simulink model "End_Angle_verification"  (R2019b)
settings: Solver=VariableStepAuto  StartTime=0.0  StopTime=10.0  RelTol=1e-3
values from neighbouring files (symbols this model uses):
  phi_d = zeros(N,1)    [parameters.m]
  phi_p = zeros(N,1)    [parameters.m]
settings Model: Creator=zceeash  LastModifiedBy=zceeash

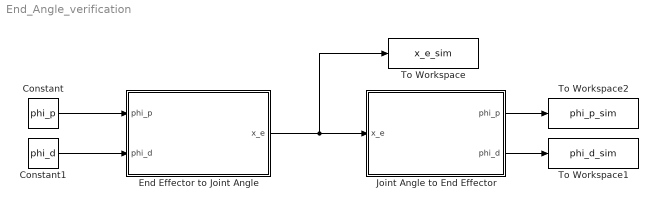
== system End_Angle_verification ==
  Constant : Constant  Value=phi_p
  Constant1 : Constant  Value=phi_d
  End Effector to Joint Angle : Subsystem
  Joint Angle to End Effector : Subsystem
  To Workspace : ToWorkspace  VariableName=x_e_sim  SaveFormat=Timeseries  SampleTime=-1
  To Workspace1 : ToWorkspace  VariableName=phi_d_sim  SaveFormat=Timeseries  SampleTime=-1
  To Workspace2 : ToWorkspace  VariableName=phi_p_sim  SaveFormat=Timeseries  SampleTime=-1
  wires:
  End Effector to Joint Angle/1(x_e) -> To Workspace/1, Joint Angle to End Effector/1(x_e)
  Joint Angle to End Effector/1(phi_p) -> To Workspace2/1
  Joint Angle to End Effector/2(phi_d) -> To Workspace1/1
  Constant/1 -> End Effector to Joint Angle/1(phi_p)
  Constant1/1 -> End Effector to Joint Angle/2(phi_d)

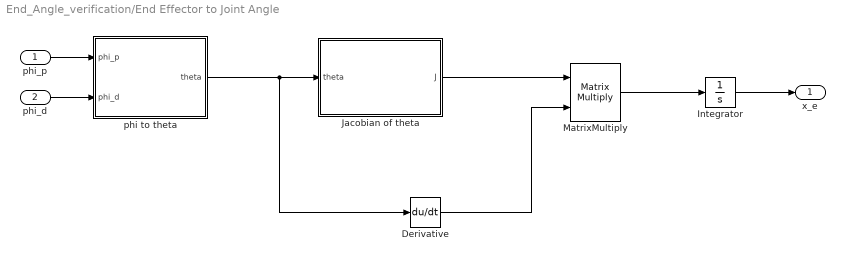
== system End_Angle_verification/End Effector to Joint Angle ==
  phi_p : Inport
  phi_d : Inport  Port=2
  Derivative : Derivative  CoefficientInTFapproximation=0
  Integrator : Integrator
  "Jacobian of theta " : MATLAB Function  TreatAsAtomicUnit=on
  MatrixMultiply : Product  Multiplication=Matrix(*)
  phi to theta : MATLAB Function  TreatAsAtomicUnit=on
  x_e : Outport
  wires:
  phi_p/1 -> phi to theta/1(phi_p)
  phi_d/1 -> phi to theta/2(phi_d)
  phi to theta/1(theta) -> Derivative/1, "Jacobian of theta "/1(theta)
  "Jacobian of theta "/1(J) -> MatrixMultiply/1
  Derivative/1 -> MatrixMultiply/2
  MatrixMultiply/1 -> Integrator/1
  Integrator/1 -> x_e/1

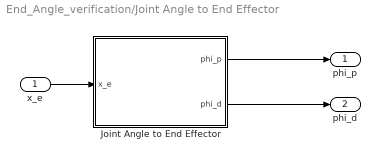
== system End_Angle_verification/Joint Angle to End Effector ==
  x_e : Inport
  Joint Angle to End Effector : MATLAB Function  TreatAsAtomicUnit=on
  phi_p : Outport
  phi_d : Outport  Port=2
  wires:
  x_e/1 -> Joint Angle to End Effector/1(x_e)
  Joint Angle to End Effector/1(phi_p) -> phi_p/1
  Joint Angle to End Effector/2(phi_d) -> phi_d/1

== matlab function End_Angle_verification/End Effector to Joint Angle/Jacobian of theta  ==
  data: theta input; J output
function J = fcn(theta)
N=9;
a=140/1000;

DH_params=[];

%Calculate D-H parameters
for i=1:N
    if rem(i,2)==0
        DH_params=[DH_params;pi pi/2 0 0; pi 0 a 0];
    else
        DH_params=[DH_params;0 pi/2 0 0; 0 0 a 0];
    end
end

A_wrt_base=eye(4);
J_w=[];
J_v=[];

%Calculate transformation matrix and then the Jacobian
for n=1:2*N
    theta_i=DH_params(n,1);
    alpha_i=DH_params(n,2);
    a_i=DH_params(n,3);
    d_i=DH_params(n,4);
    A=[cos(theta_i) -sin(theta_i)*cos(alpha_i) sin(theta_i)*sin(alpha_i) a_i*cos(theta_i);...
       sin(theta_i)  cos(theta_i)*cos(alpha_i) -cos(theta_i)*sin(alpha_i) a_i*sin(theta_i);...
                  0              sin(alpha_i)   cos(alpha_i)              d_i;...
                  0              0              0                         1];
    A_wrt_base=A;
    J_w=[J_w A_wrt_base(1:3,3)];
    J_v=[J_v A_wrt_base(1:3,3)];
end
J=[J_v J_w];

== matlab function End_Angle_verification/Joint Angle to End Effector/Joint Angle to End Effector ==
  data: x_e input; phi_p output; phi_d output
function [phi_p,phi_d] = fcn(x_e)
N=9;
a=140/1000;
d=23/2/1000;
r=20.5/1000;
error_tol=1/1000;

theta_j=zeros(2*N,1);

for i=1:N
    if rem(i,2)==0
        DH_params=[DH_params;pi pi/2 0 0; pi 0 a 0];
    else
        DH_params=[DH_params;0 pi/2 0 0; 0 0 a 0];
    end
end

x_e_j=zeros(6,1);

%Numerical iteration to find solution
for j=0:10000
   delta_x_e=x_e-x_e_j;

   if (delta_l(1)<=error_tol) && (delta_l(2)<=error_tol) && (delta_l(3)<=error_tol)
       theta=theta_j;
       break;
   end
   
   A_wrt_base=eye(4);
   J_w=[];
   J_v=[];

   for n=1:2*N
        theta_i=DH_params(n,1);
        alpha_i=DH_params(n,2);
        a_i=DH_params(n,3);
        d_i=DH_params(n,4);
        A=[cos(theta_i) -sin(theta_i)*cos(alpha_i) sin(theta_i)*sin(alpha_i) a_i*cos(theta_i);...
           sin(theta_i)  cos(theta_i)*cos(alpha_i) -cos(theta_i)*sin(alpha_i) a_i*sin(theta_i);...
                      0              sin(alpha_i)   cos(alpha_i)              d_i;...
                      0              0              0                         1];
        A_wrt_base=A;
        J_w=[J_w A_wrt_base(1:3,3)];
        J_v=[J_v A_wrt_base(1:3,3)];
   end
   
   J=[J_v J_w];
   J_inv=pinv(J);

   delta_theta= J_inv*delta_x_e;
   theta_j=theta_j+delta_theta;

   if j==10000
       theta=NaN;
   end
end
if isnan(phi_p) && isnan(phi_d)
    phi_p=theta(1:2:2*N-1);
    for n=1:N
        phi_p(n)=(-1)^(n+1)*phi_p(n);
    end
    phi_d=theta(2:2:2*N);
end
end

== matlab function End_Angle_verification/End Effector to Joint Angle/phi to theta ==
  data: phi_p input; theta output; phi_d input
function theta = fcn(phi_p,phi_d)
N=9;
%Calculate theta
theta=zeros(2*N,1);
for n=1:N
    theta(2*n-1:2*n)=[(-1)^(n+1)*phi_p;phi_d];
end
